simulink model "simulink_realworld"  (R2023b)
settings: Solver=VariableStepAuto  StartTime=0.0  StopTime=600  RelTol=1e-3
undefined symbols (not defined in the file or in its folder): gray
libraries: visiongeotforms x2, dspvision x1, deeplib x1
settings Model: SimulationMode=accelerator  Creator=Young  LastModifiedBy=Young

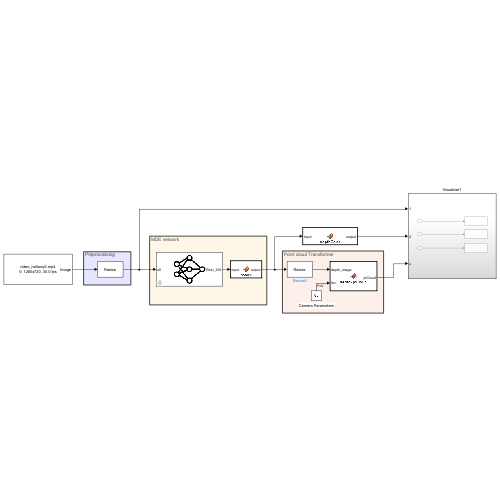
[thumbnail: Simulink's stored preview of the top-level diagram]
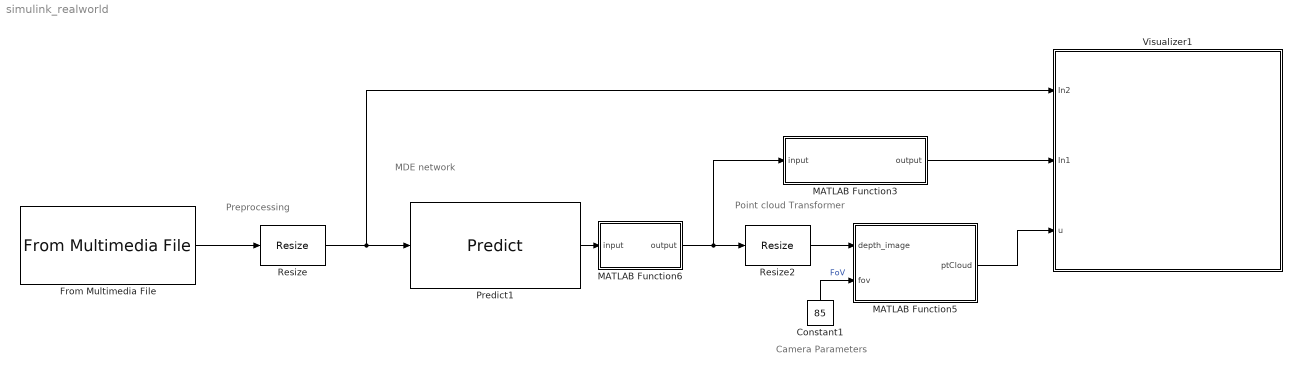
== system simulink_realworld ==
  note: Preprocessing
  note: MDE network
  note: Point cloud Transformer
  note: Camera Parameters
  Constant1 : Constant  Value=85  VectorParams1D=off
  From Multimedia File : dspvision/From Multimedia File  inputFilename=C:\Users\Young\Desktop\MATLAB_AI_COMP\test\video_hallway2.mp4  readRange=[1 Inf]  loop=on  numPlays=inf  outputStreams=Video only  videoDataType=single  audioDataType=int16  inheritSampleTime=off  userDefinedSampleTime=1/30  noAudioOutput=off  isIntensityVideo=off  fourcc=RGB  colorVideoFormat=One multidimensional signal  outputEOF=off  dataOrg=Column-major  audioFrameSize=1024  computeAudioFrameSize=off  outSamplingMode=Sample based
      settings: LibrarySourceBlock=visionsources/From Multimedia File
  MATLAB Function3 : MATLAB Function  TreatAsAtomicUnit=on
  MATLAB Function5 : MATLAB Function  TreatAsAtomicUnit=on
  MATLAB Function6 : MATLAB Function  TreatAsAtomicUnit=on
  Predict1 : deeplib/Predict  Network=Network from MAT-file  NetworkFunction=squeezenet  NetworkFilePath=C:\Users\Young\Desktop\MATLAB_AI_COMP\model\net_MDE\net_trained_20230724.mat  MiniBatchSize=128  InputDataFormats={ 'x0', 'SSCB' }  Predictions=on  Activations={}  ForceInterpretedSim=off  EnableDLNetwork=on
  Resize : visiongeotforms/Resize  specify=Number of output rows and columns  rfactor=[200 150]  outCols=25  outRows=25  outRowsCols=[384 384]  interp_method=Bilinear  antialias=on  useROI=off  roiFlag=off  roundingMode=Nearest  overflowMode=on  prodOutputMode=Binary point scaling  prodOutputWordLength=32  prodOutputFracLength=10
  Resize2 : visiongeotforms/Resize  specify=Number of output rows and columns  rfactor=[200 150]  outCols=25  outRows=25  outRowsCols=[480 640]  interp_method=Bilinear  antialias=on  useROI=off  roiFlag=off  roundingMode=Nearest  overflowMode=on  prodOutputMode=Binary point scaling  prodOutputWordLength=32  prodOutputFracLength=10
  Visualizer1 : Subsystem
  wires:
  From Multimedia File/1 -> Resize/1
  MATLAB Function3/1(output) -> Visualizer1/2(In1)
  MATLAB Function5/1(ptCloud) -> Visualizer1/3(u)
  Predict1/1 -> MATLAB Function6/1(input)
  Constant1/1 -> MATLAB Function5/2(fov)  "FoV"
  MATLAB Function6/1(output) -> Resize2/1, MATLAB Function3/1(input)
  Resize2/1 -> MATLAB Function5/1(depth_image)
  Resize/1 -> Visualizer1/1(In2), Predict1/1

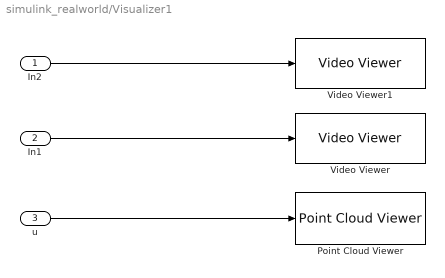
== system simulink_realworld/Visualizer1 ==
  In2 : Inport
  In1 : Inport  Port=2
  u : Inport  Port=3
  Point Cloud Viewer : PointCloudViewer  FigPos=[409.8 859.6 670.4 650.4]
  Video Viewer : VideoViewer  colormapValue=gray(256)  FigPos=[3.4 859.6 400.8 312]
  Video Viewer1 : VideoViewer  colormapValue=gray(256)  FigPos=[3.4 521.2 400.8 312]
  wires:
  In1/1 -> Video Viewer/1
  u/1 -> Point Cloud Viewer/1
  In2/1 -> Video Viewer1/1

== matlab function simulink_realworld/MATLAB Function3 ==
  data: input input; output output
function output = depthColor(input)

output = zeros([384 384 3]);

color_map = jet(256);
n_max = max(input(:));
n_min = min(input(:));

depth_data_colored = ind2rgb(uint8(256*(input - n_min)/(n_max - n_min)), color_map);
output = depth_data_colored;
end

== matlab function simulink_realworld/MATLAB Function5 ==
  data: depth_image input; fov input; ptCloud output
function ptCloud = depth2ptCloud(depth_image, fov)
%fov, depth, resolution

pixels = 640*480; % from Resolution
crop = 10;
min_distance = 1;
max_distance = 6;   

cnt = 1;
pnt_pol = zeros([pixels,3]);
%이미지 사이즈가 정해지면 mask 형식으로 간단하게 계산하는 방법도 고려해보기
for i=1+crop:480-crop %세로
    for j=1+crop:640-crop %가로
        distance = depth_image(i,j);

        %% 기준각 pi/4
        angle_vert = -((2 * (i - 1) / (480 - 1)) - 1);  % 1 -> 1, 480 -> -1  
        angle_hor = -((2 * (j - 1) / (640 - 1)) - 1);  % 1 -> 1, 640 -> -1
        theta = pi/4 + deg2rad(fov/2)*angle_hor;
        rho = distance * cos(abs(deg2rad(fov/2)*angle_hor)); 
        z = distance * sin(abs(deg2rad(fov/2)*angle_vert)) *sign(angle_vert);    % 절대값 높이 * 부호
       
        % polar to cartsian coordinate
        [x,y,z] = pol2cart(theta,rho,z);
        if distance < max_distance  && distance > min_distance
        pnt_pol(cnt,:) = [x,y,z];
        end
        cnt = cnt+1;
    end
    
end 

ptCloud = pnt_pol;

== matlab function simulink_realworld/MATLAB Function6 ==
  data: input input; output output
function output = scaler(input)

p = [0 -0.0024 8.2238];
temp = p(2)*input + p(3);
output = 0.4838*temp + 3.129;

end
